simulink model "nxtway_gs_vr"  (Simulink 7.0)
settings: Solver=ode45  StartTime=0.0  StopTime=30  MaxStep=TS  RelTol=1e-3
PreLoadFcn:
  | param_nxtway_gs
values from neighbouring files (symbols this model uses):
  pwm_gain = 1    [param_controller.m]
  pwm_offset = 0    [param_controller.m]
undefined symbols (not defined in the file or in its folder): BATTERY, BODY_HEIGHT, CAMERA_DISTANCE, CAMERA_HEIGHT, CAMERA_OFFSET, D, GP_MAX, GYRO0, MAP_WALL, R, ROTATION_X, ROTATION_Y, sigbuilder_block, START_POS, TIME_START, W
libraries: vrlib x1, simulink x1
settings Model: Creator=y_yama  LastModifiedBy=y_yama
settings DataIOCC: LimitDataPoints=off  SaveOutput=off  SignalLogging=off  SaveTime=off
settings OptimizationCC: InlineParams=on  InlineInvariantSignals=on  LifeSpan=1
settings DebuggingCC: TasksWithSamePriorityMsg=none  SigSpecEnsureSampleTimeMsg=none  IntegerOverflowMsg=none  UnknownTsInhSupMsg=none
settings HardwareCC: ProdIntDivRoundTo=Zero  ProdEndianess=LittleEndian  ProdHWDeviceType=ARM Compatible->ARM 7

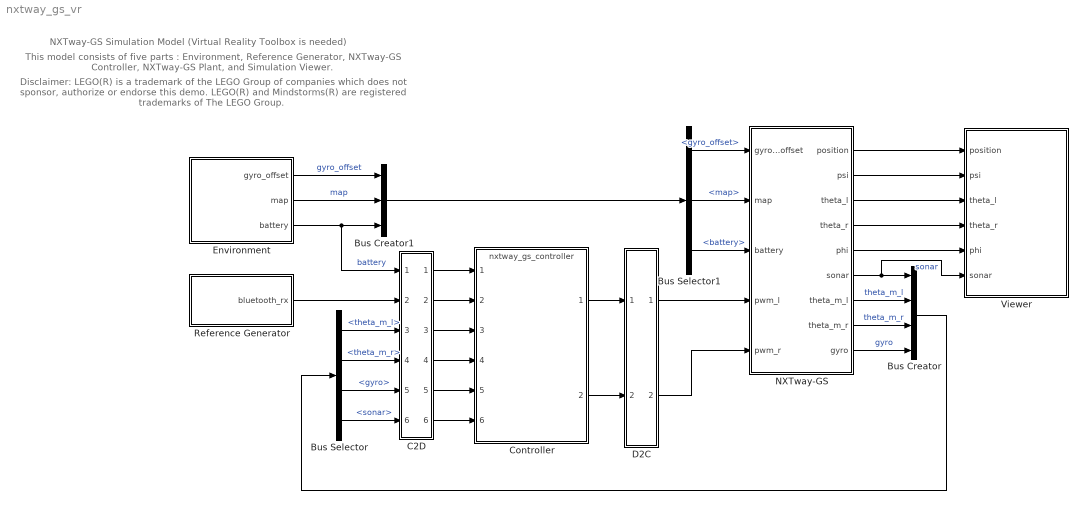
== system nxtway_gs_vr ==
  note: Disclaimer:
      | LEGO(R) is a trademark of the LEGO Group of companies which does not sponsor, authorize or endorse this demo.
      | LEGO(R) and Mindstorms(R) are registered trademarks of The LEGO Group.
  note: NXTway-GS Simulation Model (Virtual Reality Toolbox is needed)
  note: This model consists of five parts : Environment, Reference Generator, NXTway-GS Controller, NXTway-GS Plant, and Simulation Viewer.
  Bus Creator : BusCreator
  Bus Creator1 : BusCreator  Inputs=3
  Bus Selector : BusSelector  OutputSignals=theta_m_l,theta_m_r,gyro,sonar
  Bus Selector1 : BusSelector  OutputSignals=gyro_offset,map,battery
  C2D : Subsystem
      mask Display: fprintf('C2D')
  Controller : ModelReference  ModelName=nxtway_gs_controller  SimulationMode=Normal  ModelReferenceVersion=1.721  CopyOfModelName=nxtway_gs_controller
  D2C : Subsystem
      mask Display: fprintf('D2C')
  Environment : Subsystem
  NXTway-GS : Subsystem
  Reference Generator : Subsystem
  Viewer : Subsystem
  wires:
  Bus Creator/1 -> Bus Selector/1
  Environment/3(battery) -> C2D/1(In1), Bus Creator1/3  "battery"
  NXTway-GS/3(theta_l) -> Viewer/3(theta_l)
  NXTway-GS/4(theta_r) -> Viewer/4(theta_r)
  NXTway-GS/5(phi) -> Viewer/5(phi)
  Controller/1 -> D2C/1(In1)
  D2C/1(Out1) -> NXTway-GS/4(pwm_l)
  Controller/2 -> D2C/2(In2)
  D2C/2(Out2) -> NXTway-GS/5(pwm_r)
  C2D/1(Out1) -> Controller/1
  Reference Generator/1(bluetooth_rx) -> C2D/2(In2)
  C2D/2(Out2) -> Controller/2
  Bus Selector/1 -> C2D/3(In3)  "<theta_m_l>"
  Bus Selector/2 -> C2D/4(In4)  "<theta_m_r>"
  Bus Selector/3 -> C2D/5(In5)  "<gyro>"
  Bus Selector/4 -> C2D/6(In6)  "<sonar>"
  C2D/3(Out3) -> Controller/3
  C2D/4(Out4) -> Controller/4
  C2D/5(Out5) -> Controller/5
  C2D/6(Out6) -> Controller/6
  Environment/1(gyro_offset) -> Bus Creator1/1  "gyro_offset"
  Environment/2(map) -> Bus Creator1/2  "map"
  Bus Creator1/1 -> Bus Selector1/1
  Bus Selector1/1 -> NXTway-GS/1(gyro_offset)  "<gyro_offset>"
  Bus Selector1/2 -> NXTway-GS/2(map)  "<map>"
  Bus Selector1/3 -> NXTway-GS/3(battery)  "<battery>"
  NXTway-GS/2(psi) -> Viewer/2(psi)
  NXTway-GS/1(position) -> Viewer/1(position)
  NXTway-GS/6(sonar) -> Bus Creator/1, Viewer/6(sonar)  "sonar"
  NXTway-GS/7(theta_m_l) -> Bus Creator/2  "theta_m_l"
  NXTway-GS/8(theta_m_r) -> Bus Creator/3  "theta_m_r"
  NXTway-GS/9(gyro) -> Bus Creator/4  "gyro"

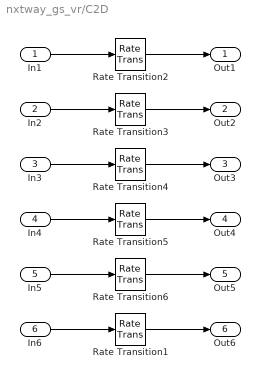
== system nxtway_gs_vr/C2D ==
  In1 : Inport  OutDataType=sfix(16)  OutScaling=2^0
  In2 : Inport  Port=2  OutDataType=sfix(16)  OutScaling=2^0
  In3 : Inport  Port=3  OutDataType=sfix(16)  OutScaling=2^0
  In4 : Inport  Port=4  OutDataType=sfix(16)  OutScaling=2^0
  In5 : Inport  Port=5  OutDataType=sfix(16)  OutScaling=2^0
  In6 : Inport  Port=6  OutDataType=sfix(16)  OutScaling=2^0
  Rate Transition{1..6} (6 alike) : RateTransition  Integrity=off  OutPortSampleTime=TS
      settings: AttributesFormatString=Ts=%<OutPortSampleTime>
  Out1 : Outport  OutDataType=sfix(16)  OutScaling=2^0
  Out2 : Outport  Port=2  OutDataType=sfix(16)  OutScaling=2^0
  Out3 : Outport  Port=3  OutDataType=sfix(16)  OutScaling=2^0
  Out4 : Outport  Port=4  OutDataType=sfix(16)  OutScaling=2^0
  Out5 : Outport  Port=5  OutDataType=sfix(16)  OutScaling=2^0
  Out6 : Outport  Port=6  OutDataType=sfix(16)  OutScaling=2^0
  wires:
  In1/1 -> Rate Transition2/1
  Rate Transition2/1 -> Out1/1
  In2/1 -> Rate Transition3/1
  In3/1 -> Rate Transition4/1
  Rate Transition3/1 -> Out2/1
  Rate Transition4/1 -> Out3/1
  In4/1 -> Rate Transition5/1
  Rate Transition5/1 -> Out4/1
  In5/1 -> Rate Transition6/1
  Rate Transition6/1 -> Out5/1
  In6/1 -> Rate Transition1/1
  Rate Transition1/1 -> Out6/1

== system nxtway_gs_vr/D2C ==
  In1 : Inport  OutDataType=sfix(16)  OutScaling=2^0
  In2 : Inport  Port=2  OutDataType=sfix(16)  OutScaling=2^0
  Rate Transition : RateTransition  Integrity=off  OutPortSampleTime=0
      settings: AttributesFormatString=Ts=%<OutPortSampleTime>
  Rate Transition1 : RateTransition  Integrity=off  OutPortSampleTime=0
      settings: AttributesFormatString=Ts=%<OutPortSampleTime>
  Out1 : Outport  SampleTime=0  OutDataType=sfix(16)  OutScaling=2^0
  Out2 : Outport  Port=2  SampleTime=0  OutDataType=sfix(16)  OutScaling=2^0
  wires:
  Rate Transition/1 -> Out1/1
  In1/1 -> Rate Transition/1
  Rate Transition1/1 -> Out2/1
  In2/1 -> Rate Transition1/1

== system nxtway_gs_vr/Environment ==
  note: Environment
  note: The charactaristics of sensors of NXTway-GS and external environment.
  Constant : Constant  Value=GYRO0  OutDataTypeMode=uint16  OutDataType=sfix(16)  OutScaling=2^0
      settings: AttributesFormatString=DataType = %<OutDataTypeStr>
  Constant1 : Constant  Value=MAP_WALL  VectorParams1D=off  OutDataTypeMode=boolean  OutDataType=sfix(16)  OutScaling=2^0
      settings: AttributesFormatString=DataType = %<OutDataTypeStr>
  Constant2 : Constant  Value=BATTERY  OutDataTypeMode=uint16  OutDataType=sfix(16)  OutScaling=2^0
      settings: AttributesFormatString=DataType = %<OutDataTypeStr>
  gyro_offset : Outport  OutDataType=sfix(16)  OutScaling=2^0
  map : Outport  Port=2  OutDataType=sfix(16)  OutScaling=2^0
  battery : Outport  Port=3  OutDataType=sfix(16)  OutScaling=2^0
  wires:
  Constant1/1 -> map/1
  Constant/1 -> gyro_offset/1
  Constant2/1 -> battery/1

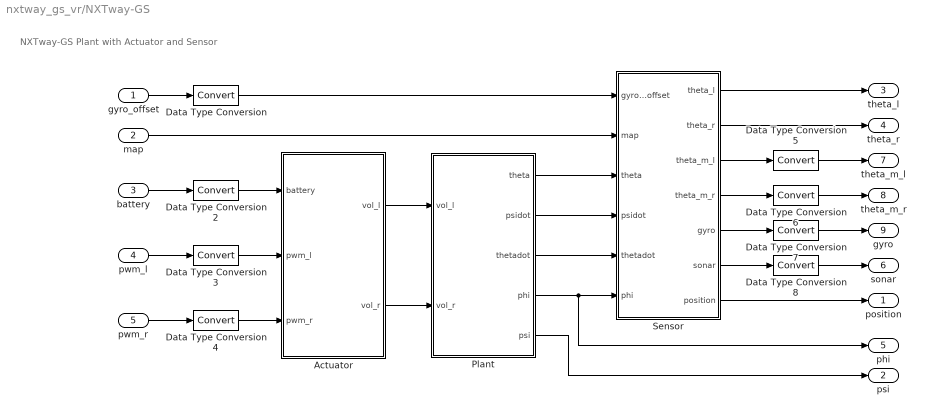
== system nxtway_gs_vr/NXTway-GS ==
  note: NXTway-GS Plant with Actuator and Sensor
  gyro_offset : Inport
  map : Inport  Port=2
  battery : Inport  Port=3
  pwm_l : Inport  Port=4
  pwm_r : Inport  Port=5
  Actuator : Subsystem
  Data Type Conversion{,2..4} (4 alike) : DataTypeConversion  OutDataTypeMode=double  OutDataType=sfix(16)  OutScaling=2^0  RndMeth=Nearest
      settings: AttributesFormatString=Round = %<RndMeth>
  Data Type Conversion5 : DataTypeConversion  OutDataTypeMode=int32  OutDataType=sfix(16)  OutScaling=2^0  RndMeth=Nearest
      settings: AttributesFormatString=Round = %<RndMeth>
  Data Type Conversion6 : DataTypeConversion  OutDataTypeMode=int32  OutDataType=sfix(16)  OutScaling=2^0  RndMeth=Nearest
      settings: AttributesFormatString=Round = %<RndMeth>
  Data Type Conversion7 : DataTypeConversion  OutDataTypeMode=uint16  OutDataType=sfix(16)  OutScaling=2^0  RndMeth=Nearest
      settings: AttributesFormatString=Round = %<RndMeth>
  Data Type Conversion8 : DataTypeConversion  OutDataTypeMode=int32  OutDataType=sfix(16)  OutScaling=2^0  RndMeth=Nearest
      settings: AttributesFormatString=Round = %<RndMeth>
  Plant : Subsystem
  Sensor : Subsystem
  position : Outport  OutDataType=sfix(16)  OutScaling=2^0
  psi : Outport  Port=2
  theta_l : Outport  Port=3
  theta_r : Outport  Port=4
  phi : Outport  Port=5
  sonar : Outport  Port=6
  theta_m_l : Outport  Port=7
  theta_m_r : Outport  Port=8
  gyro : Outport  Port=9
  wires:
  Actuator/1(vol_l) -> Plant/1(vol_l)
  Actuator/2(vol_r) -> Plant/2(vol_r)
  Plant/2(psidot) -> Sensor/4(psidot)
  Plant/1(theta) -> Sensor/3(theta)
  battery/1 -> Data Type Conversion2/1
  Sensor/1(theta_l) -> theta_l/1
  gyro_offset/1 -> Data Type Conversion/1
  Sensor/2(theta_r) -> theta_r/1
  map/1 -> Sensor/2(map)
  Sensor/3(theta_m_l) -> Data Type Conversion5/1
  Sensor/4(theta_m_r) -> Data Type Conversion6/1
  pwm_l/1 -> Data Type Conversion3/1
  Sensor/5(gyro) -> Data Type Conversion7/1
  Plant/3(thetadot) -> Sensor/5(thetadot)
  Sensor/6(sonar) -> Data Type Conversion8/1
  pwm_r/1 -> Data Type Conversion4/1
  Plant/5(psi) -> psi/1
  Data Type Conversion/1 -> Sensor/1(gyro_offset)
  Data Type Conversion2/1 -> Actuator/1(battery)
  Data Type Conversion3/1 -> Actuator/2(pwm_l)
  Data Type Conversion4/1 -> Actuator/3(pwm_r)
  Data Type Conversion5/1 -> theta_m_l/1
  Data Type Conversion6/1 -> theta_m_r/1
  Data Type Conversion7/1 -> gyro/1
  Sensor/7(position) -> position/1
  Plant/4(phi) -> Sensor/6(phi), phi/1
  Data Type Conversion8/1 -> sonar/1

== system nxtway_gs_vr/Reference Generator ==
  note: Reference Generator
  note: Reference signal generator.
  note: multiply velocity reference by -GP_MAX because negative value
      | means forward run. This is an analog stick feature of PC game pad
      | based on HID. GP_MAX is maximum of game pad input.
  Data Type Conversion1 : DataTypeConversion  OutDataTypeMode=uint8  OutDataType=sfix(16)  OutScaling=2^0  RndMeth=Nearest
      settings: AttributesFormatString=Round = %<RndMeth>
  Data Type Conversion2 : DataTypeConversion  OutDataTypeMode=uint8  OutDataType=sfix(16)  OutScaling=2^0  RndMeth=Nearest
      settings: AttributesFormatString=Round = %<RndMeth>
  Dummy Data : Constant  Value=zeros(30, 1)  OutDataTypeMode=uint8  OutDataType=sfix(16)  OutScaling=2^0
      settings: AttributesFormatString=DataType = %<OutDataTypeStr>
  Gain : Gain  Gain=-GP_MAX  ParameterDataType=sfix(16)  ParameterScaling=2^0  OutDataType=sfix(16)  OutScaling=2^0
  Gain1 : Gain  Gain=GP_MAX  ParameterDataType=sfix(16)  ParameterScaling=2^0  OutDataType=sfix(16)  OutScaling=2^0
  Mux : Mux  Inputs=3
  Signal Builder : Subsystem  Tag=STV Subsys  LoadFcn=sigbuilder_block('load');  StartFcn=sigbuilder_block('start');  StopFcn=sigbuilder_block('stop');  ClipboardFcn=sigbuilder_block('clipboard');  mask(Sigbuilder block){}
      mask help: Sigbuilder GUI
      mask init:
      | if ~strcmp(get_param(bdroot(gcbh),'SimulationStatus'),'stopped') tuvar = sigbuilder_block('maskInit'); end
      settings: CopyFcn=sigbuilder_block('copy');  DeleteFcn=sigbuilder_block('delete');  ModelCloseFcn=sigbuilder_block('modelClose');  PreSaveFcn=sigbuilder_block('preSave');  NameChangeFcn=sigbuilder_block('namechange');  OpenFcn=sigbuilder_block('open',[102.75 71.25 516 349.5 ]);  CloseFcn=sigbuilder_block('close');
      mask Display: plot(0,0,100,100,[10,10,40,40,10],[80,20,20,80,80],[40,10],[50,50], [40,27,10],[65,72,56],[40,25,25,10],[28,28,43,43]);
  bluetooth_rx : Outport  OutDataType=sfix(16)  OutScaling=2^0
  wires:
  Data Type Conversion2/1 -> Mux/1
  Data Type Conversion1/1 -> Mux/2
  Dummy Data/1 -> Mux/3
  Mux/1 -> bluetooth_rx/1
  Signal Builder/1(rdot_ref) -> Gain/1
  Gain/1 -> Data Type Conversion2/1
  Gain1/1 -> Data Type Conversion1/1
  Signal Builder/2(phidot_ref) -> Gain1/1

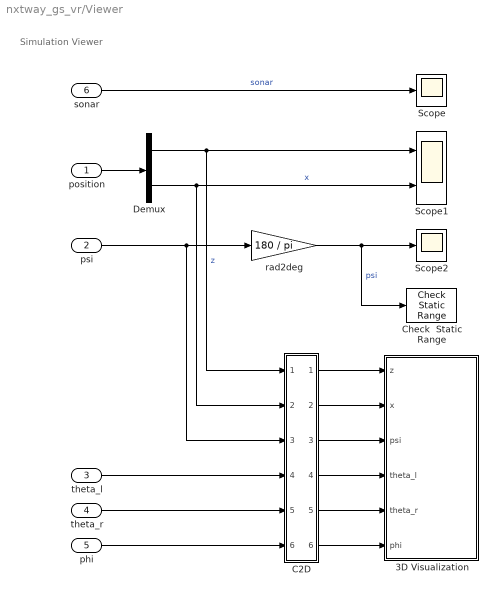
== system nxtway_gs_vr/Viewer ==
  note: Simulation Viewer
  position : Inport  OutDataType=sfix(16)  OutScaling=2^0
  psi : Inport  Port=2  OutDataType=sfix(16)  OutScaling=2^0
  theta_l : Inport  Port=3  OutDataType=sfix(16)  OutScaling=2^0
  theta_r : Inport  Port=4  OutDataType=sfix(16)  OutScaling=2^0
  phi : Inport  Port=5  OutDataType=sfix(16)  OutScaling=2^0
  sonar : Inport  Port=6  OutDataType=sfix(16)  OutScaling=2^0
  3D Visualization : Subsystem
  C2D : Subsystem
      mask Display: fprintf('C2D')
  Check  Static Range : simulink/Model Verification/Check  Static Range  Description=BODY_ANGLE_MIN <= u <= BODY_ANGLE_MAX  SystemSampleTime=-1  max=BODY_ANGLE_MAX  max_included=on  min=BODY_ANGLE_MIN  min_included=on  enabled=on  stopWhenAssertionFail=on  export=off  icon=graphic
  Demux : Demux  Outputs=2
  Scope : Scope
      settings: SaveName=ScopeData2
  Scope1 : Scope  NumInputPorts=2
      settings: YMin=-5~-5  YMax=5~5
  Scope2 : Scope
  rad2deg : Gain  Gain=180 / pi  ParameterDataType=sfix(16)  ParameterScaling=2^0  OutDataType=sfix(16)  OutScaling=2^0
  wires:
  rad2deg/1 -> Check  Static Range/1, Scope2/1  "psi"
  Demux/1 -> Scope1/1, C2D/1(In1)  "z"
  Demux/2 -> Scope1/2, C2D/2(In2)  "x"
  psi/1 -> rad2deg/1, C2D/3(In3)
  C2D/3(Out3) -> 3D Visualization/3(psi)
  theta_l/1 -> C2D/4(In4)
  theta_r/1 -> C2D/5(In5)
  phi/1 -> C2D/6(In6)
  C2D/4(Out4) -> 3D Visualization/4(theta_l)
  C2D/5(Out5) -> 3D Visualization/5(theta_r)
  C2D/6(Out6) -> 3D Visualization/6(phi)
  sonar/1 -> Scope/1  "sonar"
  position/1 -> Demux/1
  C2D/1(Out1) -> 3D Visualization/1(z)
  C2D/2(Out2) -> 3D Visualization/2(x)

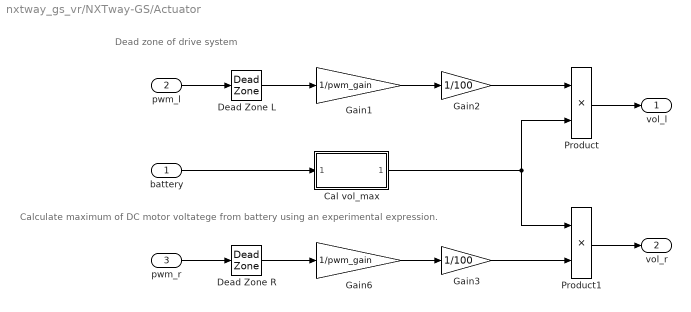
== system nxtway_gs_vr/NXTway-GS/Actuator ==
  note: Dead zone of drive system
  note: Calculate maximum of DC motor voltatege from
      | battery using an experimental expression.
  battery : Inport  OutDataType=sfix(16)  OutScaling=2^0
  pwm_l : Inport  Port=2  OutDataType=sfix(16)  OutScaling=2^0
  pwm_r : Inport  Port=3  OutDataType=sfix(16)  OutScaling=2^0
  Cal vol_max : Subsystem
  Dead Zone L : DeadZone  LowerValue=-pwm_offset  UpperValue=pwm_offset  SaturateOnIntegerOverflow=on
      settings: AttributesFormatString=start=%<LowerValue>\nend=%<UpperValue>
  Dead Zone R : DeadZone  LowerValue=-pwm_offset  UpperValue=pwm_offset  SaturateOnIntegerOverflow=on
      settings: AttributesFormatString=start=%<LowerValue>\nend=%<UpperValue>
  Gain1 : Gain  Gain=1/pwm_gain  ParameterDataType=sfix(16)  ParameterScaling=2^0  OutDataType=sfix(16)  OutScaling=2^0
  Gain2 : Gain  Gain=1/100  ParameterDataType=sfix(16)  ParameterScaling=2^0  OutDataType=sfix(16)  OutScaling=2^0
  Gain3 : Gain  Gain=1/100  ParameterDataType=sfix(16)  ParameterScaling=2^0  OutDataType=sfix(16)  OutScaling=2^0
  Gain6 : Gain  Gain=1/pwm_gain  ParameterDataType=sfix(16)  ParameterScaling=2^0  OutDataType=sfix(16)  OutScaling=2^0
  Product : Product  OutDataType=sfix(16)  OutScaling=2^0  RndMeth=Simplest
  Product1 : Product  OutDataType=sfix(16)  OutScaling=2^0  RndMeth=Simplest
  vol_l : Outport  OutDataType=sfix(16)  OutScaling=2^0
  vol_r : Outport  Port=2  OutDataType=sfix(16)  OutScaling=2^0
  wires:
  pwm_l/1 -> Dead Zone L/1
  pwm_r/1 -> Dead Zone R/1
  Gain1/1 -> Gain2/1
  Gain6/1 -> Gain3/1
  Gain2/1 -> Product/1
  Product/1 -> vol_l/1
  Gain3/1 -> Product1/2
  Product1/1 -> vol_r/1
  Dead Zone L/1 -> Gain1/1
  Dead Zone R/1 -> Gain6/1
  Cal vol_max/1(vol_max) -> Product/2, Product1/1
  battery/1 -> Cal vol_max/1(battery)

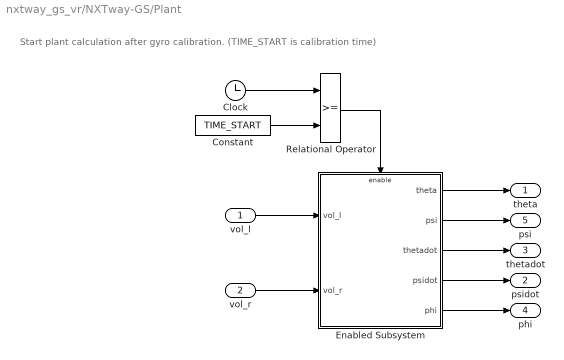
== system nxtway_gs_vr/NXTway-GS/Plant ==
  note: Start plant calculation after gyro calibration.
      | (TIME_START is calibration time)
  vol_l : Inport
  vol_r : Inport  Port=2
  Clock : Clock
  Constant : Constant  Value=TIME_START  OutDataTypeMode=double  OutDataType=sfix(16)  OutScaling=2^0
      settings: AttributesFormatString=DataType = %<OutDataTypeStr>
  Enabled Subsystem : Subsystem  TreatAsAtomicUnit=on
  Relational Operator : RelationalOperator  LogicOutDataTypeMode=boolean
  theta : Outport
  psidot : Outport  Port=2
  thetadot : Outport  Port=3
  phi : Outport  Port=4
  psi : Outport  Port=5
  wires:
  vol_l/1 -> Enabled Subsystem/1(vol_l)
  vol_r/1 -> Enabled Subsystem/2(vol_r)
  Relational Operator/1 -> Enabled Subsystem/Enable
  Clock/1 -> Relational Operator/1
  Constant/1 -> Relational Operator/2
  Enabled Subsystem/1(theta) -> theta/1
  Enabled Subsystem/3(thetadot) -> thetadot/1
  Enabled Subsystem/2(psi) -> psi/1
  Enabled Subsystem/5(phi) -> phi/1
  Enabled Subsystem/4(psidot) -> psidot/1

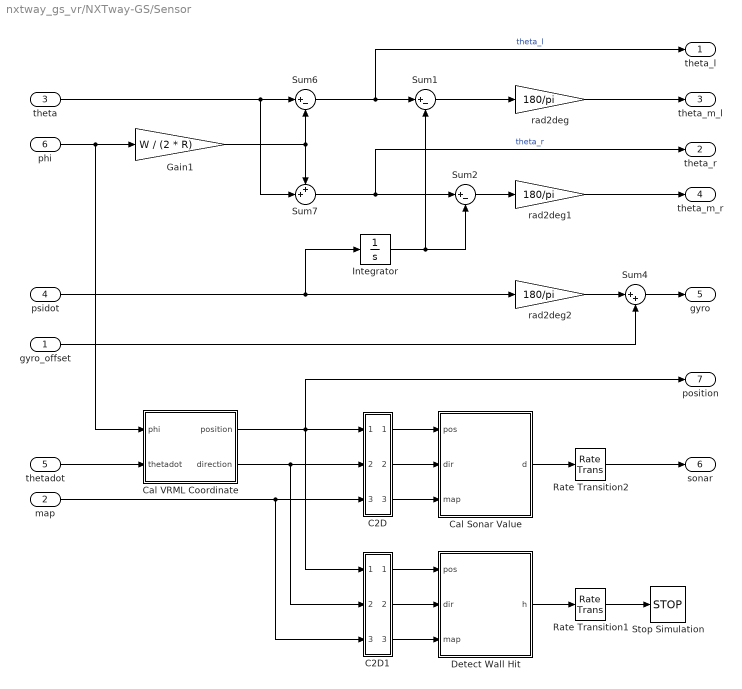
== system nxtway_gs_vr/NXTway-GS/Sensor ==
  gyro_offset : Inport  OutDataType=sfix(16)  OutScaling=2^0
  map : Inport  Port=2  OutDataType=sfix(16)  OutScaling=2^0
  theta : Inport  Port=3  OutDataType=sfix(16)  OutScaling=2^0
  psidot : Inport  Port=4  OutDataType=sfix(16)  OutScaling=2^0
  thetadot : Inport  Port=5  OutDataType=sfix(16)  OutScaling=2^0
  phi : Inport  Port=6  OutDataType=sfix(16)  OutScaling=2^0
  C2D : Subsystem
      mask Display: fprintf('C2D')
  C2D1 : Subsystem
      mask Display: fprintf('C2D')
  Cal Sonar Value : Stateflow chart
  Cal VRML Coordinate : Subsystem
  Detect Wall Hit : Stateflow chart
  Gain1 : Gain  Gain=W / (2 * R)  ParameterDataType=sfix(16)  ParameterScaling=2^0  OutDataType=sfix(16)  OutScaling=2^0
  Integrator : Integrator
  Rate Transition1 : RateTransition  Integrity=off  OutPortSampleTime=0
      settings: AttributesFormatString=Ts=%<OutPortSampleTime>
  Rate Transition2 : RateTransition  Integrity=off  OutPortSampleTime=0
      settings: AttributesFormatString=Ts=%<OutPortSampleTime>
  Stop Simulation : Stop
  Sum1 : Sum  Inputs=|+-  OutDataType=sfix(16)  OutScaling=2^0
  Sum2 : Sum  Inputs=|+-  OutDataType=sfix(16)  OutScaling=2^0
  Sum4 : Sum  Inputs=|++  OutDataType=sfix(16)  OutScaling=2^0
  Sum6 : Sum  Inputs=|+-  OutDataType=sfix(16)  OutScaling=2^0
  Sum7 : Sum  Inputs=++|  OutDataType=sfix(16)  OutScaling=2^0
  rad2deg : Gain  Gain=180/pi  ParameterDataType=sfix(16)  ParameterScaling=2^0  OutDataType=sfix(16)  OutScaling=2^0
  rad2deg1 : Gain  Gain=180/pi  ParameterDataType=sfix(16)  ParameterScaling=2^0  OutDataType=sfix(16)  OutScaling=2^0
  rad2deg2 : Gain  Gain=180/pi  ParameterDataType=sfix(16)  ParameterScaling=2^0  OutDataType=sfix(16)  OutScaling=2^0
  theta_l : Outport  OutDataType=sfix(16)  OutScaling=2^0
  theta_r : Outport  Port=2  OutDataType=sfix(16)  OutScaling=2^0
  theta_m_l : Outport  Port=3  OutDataType=sfix(16)  OutScaling=2^0
  theta_m_r : Outport  Port=4  OutDataType=sfix(16)  OutScaling=2^0
  gyro : Outport  Port=5  OutDataType=sfix(16)  OutScaling=2^0
  sonar : Outport  Port=6  OutDataType=sfix(16)  OutScaling=2^0
  position : Outport  Port=7  OutDataType=sfix(16)  OutScaling=2^0
  wires:
  Integrator/1 -> Sum2/2, Sum1/2
  Sum4/1 -> gyro/1
  gyro_offset/1 -> Sum4/2
  Sum7/1 -> Sum2/1, theta_r/1  "theta_r"
  rad2deg2/1 -> Sum4/1
  theta/1 -> Sum7/2, Sum6/1
  phi/1 -> Gain1/1, Cal VRML Coordinate/1(phi)
  Gain1/1 -> Sum7/1, Sum6/2
  Sum1/1 -> rad2deg/1
  psidot/1 -> Integrator/1, rad2deg2/1
  Sum2/1 -> rad2deg1/1
  rad2deg/1 -> theta_m_l/1
  rad2deg1/1 -> theta_m_r/1
  Sum6/1 -> Sum1/1, theta_l/1  "theta_l"
  thetadot/1 -> Cal VRML Coordinate/2(thetadot)
  Cal Sonar Value/1(d) -> Rate Transition2/1
  Rate Transition2/1 -> sonar/1
  Cal VRML Coordinate/1(position) -> position/1, C2D/1(In1), C2D1/1(In1)
  map/1 -> C2D1/3(In3), C2D/3(In3)
  C2D/3(Out3) -> Cal Sonar Value/3(map)
  C2D/1(Out1) -> Cal Sonar Value/1(pos)
  Cal VRML Coordinate/2(direction) -> C2D/2(In2), C2D1/2(In2)
  C2D/2(Out2) -> Cal Sonar Value/2(dir)
  Detect Wall Hit/1(h) -> Rate Transition1/1
  C2D1/1(Out1) -> Detect Wall Hit/1(pos)
  C2D1/2(Out2) -> Detect Wall Hit/2(dir)
  C2D1/3(Out3) -> Detect Wall Hit/3(map)
  Rate Transition1/1 -> Stop Simulation/1

== system nxtway_gs_vr/Reference Generator/Signal Builder ==
  Demux : Demux  Tag=STV Demux  Outputs=2
  FromWs : FromWorkspace  Tag=STV FromWs  VariableName=tuvar  SampleTime=0  SigBuilderData=DataTag0  VnvData=DataTag1
      SigBuilderData=|
      | channels(1).label = 'rdot_ref'
      | channels(1).allXData = {[0 25], [0 5 5 10 10 15 15 20 20 25], [0 10 10 15 15 20 20 25], [0 6.4 6.4 25]}
      | channels(1).allYData = {[0 0], [0 0 1 1 0 0 -1 -1 0 0], [0 0 1 1 0 0 1 1], [0 0 1 1]}
      | channels(2).label = 'phidot_ref'
      | channels(2).allXData = {[0 25], [0 25], [0 5 5 10 10 15 15 20 20 25], [0 5 5 6.4 6.4 15 20 25]}
      | channels(2).allYData = {[0 0], [0 0], [0 0 1 1 0 0 -1 -1 0 0], [0 0 -1 -1 0 0 0 0]}
      | common.afterFinalStr = 'Extrapolate'
      | common.sampleTime = 0
      | dataSet(1).timeRange = [0 25]
      | dataSet(1).name = 'Stand'
      | dataSet(2).timeRange = [0 25]
      | dataSet(2).name = 'Forward & Back'
      | dataSet(3).timeRange = [0 25]
      | dataSet(3).name = 'Turn'
      | dataSet(4).timeRange = [0 25]
      | dataSet(4).name = 'Approach Wall'
  rdot_ref : Outport  Tag=STV Outport  OutDataType=sfix(16)  OutScaling=2^0
  phidot_ref : Outport  Tag=STV Outport  Port=2
  wires:
  FromWs/1 -> Demux/1
  Demux/1 -> rdot_ref/1
  Demux/2 -> phidot_ref/1

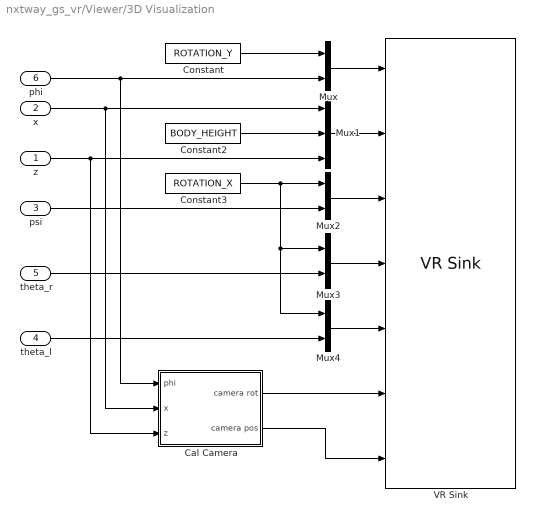
== system nxtway_gs_vr/Viewer/3D Visualization ==
  z : Inport  OutDataType=sfix(16)  OutScaling=2^0
  x : Inport  Port=2  OutDataType=sfix(16)  OutScaling=2^0
  psi : Inport  Port=3  OutDataType=sfix(16)  OutScaling=2^0
  theta_l : Inport  Port=4  OutDataType=sfix(16)  OutScaling=2^0
  theta_r : Inport  Port=5  OutDataType=sfix(16)  OutScaling=2^0
  phi : Inport  Port=6  OutDataType=sfix(16)  OutScaling=2^0
  Cal Camera : Subsystem
  Constant : Constant  Value=ROTATION_Y  OutDataTypeMode=double  OutDataType=sfix(16)  OutScaling=2^0
      settings: AttributesFormatString=DataType = %<OutDataTypeStr>
  Constant2 : Constant  Value=BODY_HEIGHT  OutDataTypeMode=double  OutDataType=sfix(16)  OutScaling=2^0
      settings: AttributesFormatString=DataType = %<OutDataTypeStr>
  Constant3 : Constant  Value=ROTATION_X  OutDataTypeMode=double  OutDataType=sfix(16)  OutScaling=2^0
      settings: AttributesFormatString=DataType = %<OutDataTypeStr>
  Mux{,2..4} (4 alike) : Mux  Inputs=2
  Mux1 : Mux  Inputs=3
  VR Sink : vrlib/VR Sink  SampleTime=-1  ViewEnable=on  RemoteChange=off  RemoteView=off  FieldsWritten=NXT.rotation.4.1.double#NXT.translation.3.1.double#NXT_body.rotation.4.1.double#NXT_tyreR.rotation.4.1.double#NXT_tyreL.rotation.4.1.double#Camera.rotation.4.1.double#Camera.translation.3.1.double  WorldFileName=vrnxtwaytrack.wrl  AutoView=on  VideoDimensions=[]  FigureProperties="{'Position', 'Name', 'Viewpoint', 'CameraBound', 'CameraDirection', 'CameraPosition', 'CameraUpVector', 'ZoomFactor', 'Antialiasing', 'Headlight', 'Lighting', 'NavPanel', 'StatusBar', 'ToolBar', 'Textures', 'Transparency', 'Wireframe', 'NavZones', 'NavMode', 'NavSpeed', 'Record2DCompressMethod', 'Record2DCompressQuality', 'Record2D', 'Record2DFileName', 'Record2DFPS'; [6.6100000000000000e+002  2.2300000000000000e+002  5.7600000000000000e+002  3.8000000000000000e+002], '', 'Chaser view', 'on', [0.0000000000000000e+000  0.0000000000000000e+000 -1.0000000000000000e+000], [0.0000000000000000e+000  0.0000000000000000e+000  0.0000000000000000e+000], [0.0000000000000000e+000  1.0000000000000000e+000  0.0000000000000000e+000], [1.0000000000000000e+000], 'off', 'off', 'on', 'halfbar', 'on', 'on', 'on', 'on', 'off', 'off', 'walk', 'normal', 'auto', [7.5000000000000000e+001], 'off', '%f_anim_%n.avi', [1.5000000000000000e+001]}"
  wires:
  theta_l/1 -> Mux4/2
  theta_r/1 -> Mux3/2
  psi/1 -> Mux2/2
  Constant3/1 -> Mux4/1, Mux3/1, Mux2/1
  z/1 -> Mux1/3, Cal Camera/3(z)
  Constant2/1 -> Mux1/2
  x/1 -> Mux1/1, Cal Camera/2(x)
  Constant/1 -> Mux/1
  phi/1 -> Mux/2, Cal Camera/1(phi)
  Mux/1 -> VR Sink/1
  Mux1/1 -> VR Sink/2
  Mux2/1 -> VR Sink/3
  Mux3/1 -> VR Sink/4
  Mux4/1 -> VR Sink/5
  Cal Camera/2(camera pos) -> VR Sink/7
  Cal Camera/1(camera rot) -> VR Sink/6

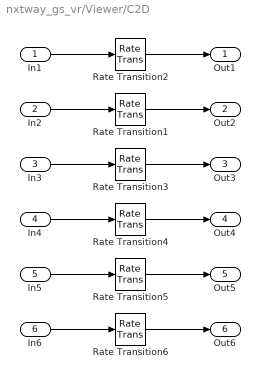
== system nxtway_gs_vr/Viewer/C2D ==
  In1 : Inport  OutDataType=sfix(16)  OutScaling=2^0
  In2 : Inport  Port=2  OutDataType=sfix(16)  OutScaling=2^0
  In3 : Inport  Port=3  OutDataType=sfix(16)  OutScaling=2^0
  In4 : Inport  Port=4  OutDataType=sfix(16)  OutScaling=2^0
  In5 : Inport  Port=5  OutDataType=sfix(16)  OutScaling=2^0
  In6 : Inport  Port=6  OutDataType=sfix(16)  OutScaling=2^0
  Rate Transition{1..6} (6 alike) : RateTransition  Integrity=off  OutPortSampleTime=TS_VR
      settings: AttributesFormatString=Ts=%<OutPortSampleTime>
  Out1 : Outport  OutDataType=sfix(16)  OutScaling=2^0
  Out2 : Outport  Port=2  OutDataType=sfix(16)  OutScaling=2^0
  Out3 : Outport  Port=3  OutDataType=sfix(16)  OutScaling=2^0
  Out4 : Outport  Port=4  OutDataType=sfix(16)  OutScaling=2^0
  Out5 : Outport  Port=5  OutDataType=sfix(16)  OutScaling=2^0
  Out6 : Outport  Port=6  OutDataType=sfix(16)  OutScaling=2^0
  wires:
  Rate Transition6/1 -> Out6/1
  In6/1 -> Rate Transition6/1
  Rate Transition5/1 -> Out5/1
  In5/1 -> Rate Transition5/1
  Rate Transition4/1 -> Out4/1
  In4/1 -> Rate Transition4/1
  Rate Transition3/1 -> Out3/1
  Rate Transition1/1 -> Out2/1
  In3/1 -> Rate Transition3/1
  In2/1 -> Rate Transition1/1
  Rate Transition2/1 -> Out1/1
  In1/1 -> Rate Transition2/1

== system nxtway_gs_vr/NXTway-GS/Actuator/Cal vol_max ==
  battery : Inport
  Constant : Constant  Value=0.625  OutDataTypeMode=double  OutDataType=sfix(16)  OutScaling=2^0
      settings: AttributesFormatString=DataType = %<OutDataTypeStr>
  Gain3 : Gain  Gain=0.001089  ParameterDataType=sfix(16)  ParameterScaling=2^0  OutDataType=sfix(16)  OutScaling=2^0
  Sum2 : Sum  Inputs=|+-  OutDataType=sfix(16)  OutScaling=2^0
  vol_max : Outport
  wires:
  battery/1 -> Gain3/1
  Gain3/1 -> Sum2/1
  Sum2/1 -> vol_max/1
  Constant/1 -> Sum2/2

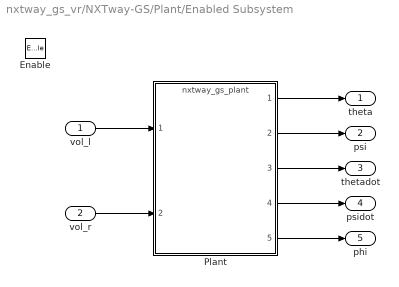
== system nxtway_gs_vr/NXTway-GS/Plant/Enabled Subsystem ==
  vol_l : Inport
  vol_r : Inport  Port=2
  Enable : EnablePort
  Plant : ModelReference  ModelName=nxtway_gs_plant  SimulationMode=Normal  ModelReferenceVersion=1.41  CopyOfModelName=nxtway_gs_plant
  theta : Outport  InitialOutput=0
  psi : Outport  Port=2  InitialOutput=0
  thetadot : Outport  Port=3  InitialOutput=0
  psidot : Outport  Port=4  InitialOutput=0
  phi : Outport  Port=5  InitialOutput=0
  wires:
  vol_l/1 -> Plant/1
  vol_r/1 -> Plant/2
  Plant/1 -> theta/1
  Plant/2 -> psi/1
  Plant/3 -> thetadot/1
  Plant/4 -> psidot/1
  Plant/5 -> phi/1

== system nxtway_gs_vr/NXTway-GS/Sensor/C2D ==
  In1 : Inport  OutDataType=sfix(16)  OutScaling=2^0
  In2 : Inport  Port=2  OutDataType=sfix(16)  OutScaling=2^0
  In3 : Inport  Port=3  OutDataType=sfix(16)  OutScaling=2^0
  Rate Transition1 : RateTransition  Integrity=off  OutPortSampleTime=TS_SONAR
      settings: AttributesFormatString=Ts=%<OutPortSampleTime>
  Rate Transition2 : RateTransition  Integrity=off  OutPortSampleTime=TS_SONAR
      settings: AttributesFormatString=Ts=%<OutPortSampleTime>
  Rate Transition3 : RateTransition  Integrity=off  OutPortSampleTime=TS_SONAR
      settings: AttributesFormatString=Ts=%<OutPortSampleTime>
  Out1 : Outport  OutDataType=sfix(16)  OutScaling=2^0
  Out2 : Outport  Port=2  OutDataType=sfix(16)  OutScaling=2^0
  Out3 : Outport  Port=3  OutDataType=sfix(16)  OutScaling=2^0
  wires:
  Rate Transition3/1 -> Out3/1
  Rate Transition1/1 -> Out2/1
  In3/1 -> Rate Transition3/1
  In2/1 -> Rate Transition1/1
  Rate Transition2/1 -> Out1/1
  In1/1 -> Rate Transition2/1

== system nxtway_gs_vr/NXTway-GS/Sensor/C2D1 ==
  In1 : Inport  OutDataType=sfix(16)  OutScaling=2^0
  In2 : Inport  Port=2  OutDataType=sfix(16)  OutScaling=2^0
  In3 : Inport  Port=3  OutDataType=sfix(16)  OutScaling=2^0
  Rate Transition1 : RateTransition  Integrity=off  OutPortSampleTime=TS_WALL
      settings: AttributesFormatString=Ts=%<OutPortSampleTime>
  Rate Transition2 : RateTransition  Integrity=off  OutPortSampleTime=TS_WALL
      settings: AttributesFormatString=Ts=%<OutPortSampleTime>
  Rate Transition3 : RateTransition  Integrity=off  OutPortSampleTime=TS_WALL
      settings: AttributesFormatString=Ts=%<OutPortSampleTime>
  Out1 : Outport  OutDataType=sfix(16)  OutScaling=2^0
  Out2 : Outport  Port=2  OutDataType=sfix(16)  OutScaling=2^0
  Out3 : Outport  Port=3  OutDataType=sfix(16)  OutScaling=2^0
  wires:
  In1/1 -> Rate Transition2/1
  Rate Transition2/1 -> Out1/1
  In2/1 -> Rate Transition1/1
  In3/1 -> Rate Transition3/1
  Rate Transition1/1 -> Out2/1
  Rate Transition3/1 -> Out3/1

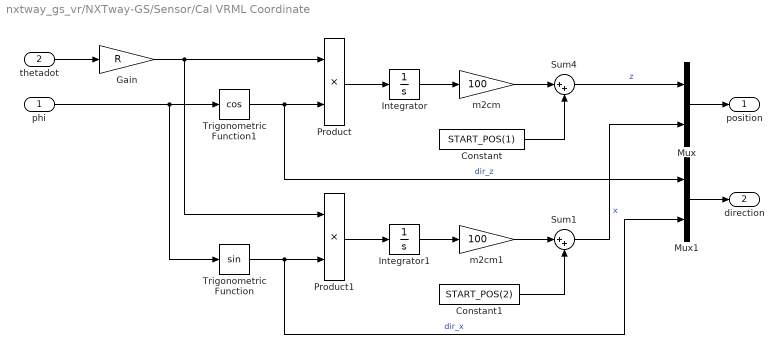
== system nxtway_gs_vr/NXTway-GS/Sensor/Cal VRML Coordinate ==
  phi : Inport
  thetadot : Inport  Port=2
  Constant : Constant  Value=START_POS(1)  OutDataTypeMode=double  OutDataType=sfix(16)  OutScaling=2^0
      settings: AttributesFormatString=DataType = %<OutDataTypeStr>
  Constant1 : Constant  Value=START_POS(2)  OutDataTypeMode=double  OutDataType=sfix(16)  OutScaling=2^0
      settings: AttributesFormatString=DataType = %<OutDataTypeStr>
  Gain : Gain  Gain=R  ParameterDataType=sfix(16)  ParameterScaling=2^0  OutDataType=sfix(16)  OutScaling=2^0
  Integrator : Integrator
  Integrator1 : Integrator
  Mux : Mux  Inputs=2
  Mux1 : Mux  Inputs=2
  Product : Product  OutDataType=sfix(16)  OutScaling=2^0  RndMeth=Simplest
  Product1 : Product  OutDataType=sfix(16)  OutScaling=2^0  RndMeth=Simplest
  Sum1 : Sum  Inputs=|++  OutDataType=sfix(16)  OutScaling=2^0
  Sum4 : Sum  Inputs=|++  OutDataType=sfix(16)  OutScaling=2^0
  Trigonometric Function : Trigonometry
  Trigonometric Function1 : Trigonometry  Operator=cos
  m2cm : Gain  Gain=100  ParameterDataType=sfix(16)  ParameterScaling=2^0  OutDataType=sfix(16)  OutScaling=2^0
  m2cm1 : Gain  Gain=100  ParameterDataType=sfix(16)  ParameterScaling=2^0  OutDataType=sfix(16)  OutScaling=2^0
  position : Outport
  direction : Outport  Port=2
  wires:
  Product1/1 -> Integrator1/1
  Trigonometric Function/1 -> Product1/2, Mux1/2  "dir_x"
  Product/1 -> Integrator/1
  Trigonometric Function1/1 -> Product/2, Mux1/1  "dir_z"
  thetadot/1 -> Gain/1
  phi/1 -> Trigonometric Function1/1, Trigonometric Function/1
  Integrator/1 -> m2cm/1
  Integrator1/1 -> m2cm1/1
  Gain/1 -> Product1/1, Product/1
  m2cm/1 -> Sum4/1
  Sum4/1 -> Mux/1  "z"
  Constant/1 -> Sum4/2
  m2cm1/1 -> Sum1/1
  Constant1/1 -> Sum1/2
  Sum1/1 -> Mux/2  "x"
  Mux/1 -> position/1
  Mux1/1 -> direction/1

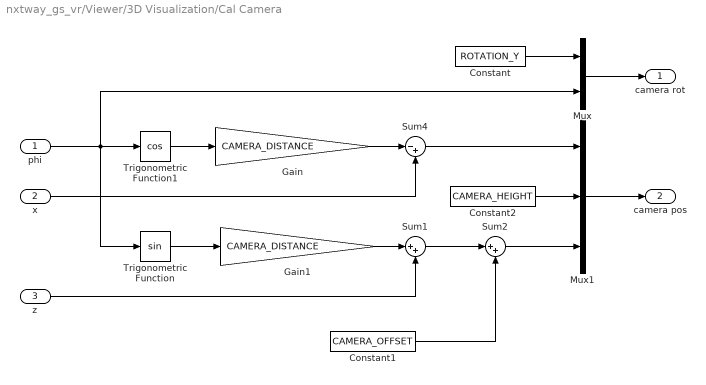
== system nxtway_gs_vr/Viewer/3D Visualization/Cal Camera ==
  phi : Inport  OutDataType=sfix(16)  OutScaling=2^0
  x : Inport  Port=2  OutDataType=sfix(16)  OutScaling=2^0
  z : Inport  Port=3  OutDataType=sfix(16)  OutScaling=2^0
  Constant : Constant  Value=ROTATION_Y  OutDataType=sfix(16)  OutScaling=2^0
      settings: AttributesFormatString=DataType = %<OutDataTypeStr>
  Constant1 : Constant  Value=CAMERA_OFFSET  OutDataType=sfix(16)  OutScaling=2^0
      settings: AttributesFormatString=DataType = %<OutDataTypeStr>
  Constant2 : Constant  Value=CAMERA_HEIGHT  OutDataType=sfix(16)  OutScaling=2^0
      settings: AttributesFormatString=DataType = %<OutDataTypeStr>
  Gain : Gain  Gain=CAMERA_DISTANCE  ParameterDataType=sfix(16)  ParameterScaling=2^0  OutDataType=sfix(16)  OutScaling=2^0
  Gain1 : Gain  Gain=CAMERA_DISTANCE  ParameterDataType=sfix(16)  ParameterScaling=2^0  OutDataType=sfix(16)  OutScaling=2^0
  Mux : Mux  Inputs=2
  Mux1 : Mux  Inputs=3
  Sum1 : Sum  Inputs=|++  OutDataType=sfix(16)  OutScaling=2^0
  Sum2 : Sum  Inputs=|++  OutDataType=sfix(16)  OutScaling=2^0
  Sum4 : Sum  Inputs=|-+  OutDataType=sfix(16)  OutScaling=2^0
  Trigonometric Function : Trigonometry
  Trigonometric Function1 : Trigonometry  Operator=cos
  camera rot : Outport  OutDataType=sfix(16)  OutScaling=2^0
  camera pos : Outport  Port=2  OutDataType=sfix(16)  OutScaling=2^0
  wires:
  Constant2/1 -> Mux1/2
  Sum4/1 -> Mux1/1
  Mux1/1 -> camera pos/1
  phi/1 -> Trigonometric Function1/1, Trigonometric Function/1, Mux/2
  Trigonometric Function1/1 -> Gain/1
  z/1 -> Sum1/2
  Gain1/1 -> Sum1/1
  Trigonometric Function/1 -> Gain1/1
  Gain/1 -> Sum4/1
  x/1 -> Sum4/2
  Constant/1 -> Mux/1
  Mux/1 -> camera rot/1
  Sum1/1 -> Sum2/1
  Sum2/1 -> Mux1/3
  Constant1/1 -> Sum2/2

== matlab function NXTway-GS/Sensor/Detect Wall Hit ==
  data: pos input inherited; h output boolean; dir input inherited; map input inherited; D parameter inherited; W parameter inherited
function h = hit_wall(pos, dir, map, D, W)
% Detect if NXTway hits the wall
% Inputs:
%   pos    : NXTway position ([z, x]) [cm]
%   dir    : NXTway direction vector ([z, x]) [cm]
%   map    : wall map
% Outputs:
%   h      : wall hit flag

eml.extrinsic('errordlg');

h = false;
posh = zeros(6, 2);
[rows, cols] = size(map);
tmp1 = (D / 2) * dir;
tmp2 = (W / 2) * [dir(2), -dir(1)];

posh(2, :) = pos + tmp1;
posh(5, :) = pos - tmp1;
posh(1, :) = posh(2, :) + tmp2;
posh(6, :) = posh(5, :) + tmp2;
posh(3, :) = posh(2, :) - tmp2;
posh(4, :) = posh(5, :) - tmp2;

for n = 1:6
	if posh(n, 1) <= 0 || posh(n, 1) >= rows ...
			|| posh(n, 2) <= 0 || posh(n, 2) >= cols
		% outside map
		h = false;
	else
		% inside map
		h = iswall(posh(n, :), map);
		if h == true
			errordlg('NXTway-GS Hits Wall !', 'Wall Hit Detection');
			break;
		end
	end
end

== matlab function NXTway-GS/Sensor/Cal Sonar Value ==
  data: pos input inherited; dir input inherited; d output inherited; map input inherited
function d = cal_sonar(pos, dir, map)
% Calcurate sonar value (distance)
% Inputs:
%   pos    : NXTway position ([z, x]) [cm]
%   dir    : NXTway direction vector ([z, x]) [cm]
%   map    : wall map
% Outputs:
%   d      : sonar value (distance) [cm]

d = 1;
[rows, cols] = size(map);

while d < 255
	posd = pos + d * dir;
	if posd(1) <= 0 || posd(1) >= rows ...
			|| posd(2) <= 0 || posd(2) >= cols
		% outside map
		d = 255;
	else
		% inside map
		flag = iswall(posd, map);
		if flag == true
			break;
		else
			d = d + 1;
		end
	end
end
